simulink library "ThermalNodeTHB"  (R2018b)
settings: Solver=ode45  StartTime=0.0  StopTime=10.0  RelTol=1e-3  EnableMultiTasking=on
libraries: carnot x2
settings Model: Creator=Hafner  LastModifiedBy=drhf
settings DataIOCC: LimitDataPoints=on  SaveFormat=Array  SignalLoggingSaveFormat=ModelDataLogs
settings OptimizationCC: ExpressionDepthLimit=2147483647  LifeSpan=inf
settings DebuggingCC: UnderspecifiedInitializationDetection=Classic  MergeDetectMultiDrivingBlocksExec=none  SolverPrmCheckMsg=warning  FcnCallInpInsideContextMsg=warning  StateNameClashWarn=warning  SFUnexpectedBacktrackingDiag=warning  SFNoUnconditionalDefaultTransitionDiag=warning  SFExecutionAtInitializationDiag=none
settings HardwareCC: ProdBitPerPointer=32  ProdBitPerSizeT=32  ProdBitPerPtrDiffT=32  ProdLargestAtomicFloat=None  ProdIntDivRoundTo=Undefined  ProdEndianess=Unspecified  ProdWordSize=32  ProdHWDeviceType=32-bit Generic
settings ModelReferenceCC: PropagateSignalLabelsOutOfModel=off
settings SFSimCC: SimUseLocalCustomCode=off
settings RTWCC: RTWUseLocalCustomCode=off
settings CodeAppCC: StateflowObjectComments=on
settings GRTTargetCC: TargetLangStandard=C89/C90 (ANSI)  GeneratePreprocessorConditionals=Disable all  CombineOutputUpdateFcns=off  GRTInterface=on
settings ConfigComp: CovMetricSettings=dw  CovHtmlReporting=on  CovSaveCumulativeToWorkspaceVar=on  CovSaveSingleToWorkspaceVar=on  CovExternalEMLEnable=off

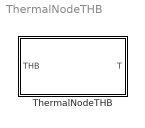
== system ThermalNodeTHB ==
  ThermalNodeTHB : Subsystem  mask(Thermal Node){UA=1, mcp=4182, Tini=20}
      mask prompts: UA "UA: thermal loss coefficient in W/K"; mcp "mcp: thermal capacity of the node in J/K"; Tini "Ambient temperature for losses (and initial Temp.) in °C"
      mask help: Thermal node with the THB as input.
      mask Help: web(fullfile(path_carnot('help'),'Thermal_Node.html'),'-helpbrowser')
      mask TypeOptions UA: Thermal_Node/UA
      mask TypeOptions mcp: Thermal_Node/mcp
      mask TypeOptions Tini: Tamb/Value
      mask Display: plot(-20,0,120,100,[10,70,70,10,10],[10,10,70,70,10],[70,90,90,30,10],[10,30,90,90,70],[90,70],[90,70],[50,30],[60,60],[40,40],[30,60])

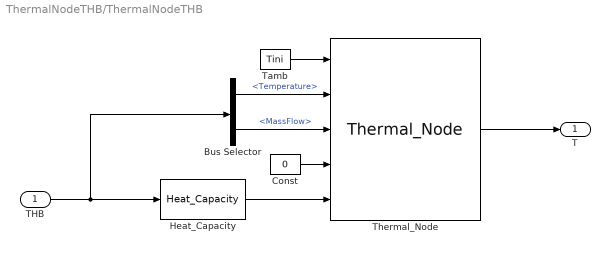
== system ThermalNodeTHB/ThermalNodeTHB ==
  THB : Inport
  Bus Selector : BusSelector  OutputSignals=Temperature,MassFlow
  Const : Constant  Value=0
  Heat_Capacity : carnot/Basic/Material_Properties/Heat_Capacity  VariantControl=CarlibClassic  INPUTARGUMENTS=THB  DEBUGLEVEL=DEBUGLEVEL  MAXTOTALWARNINGS=inf  MAXCONSECUTIVEWARNINGS=inf  WRITETOFILE=0  FILENAME='errors.txt'
      settings: SourceProductName=Carnot
  Tamb : Constant  Value=Tini
  Thermal_Node : carnot/Basic/Thermal_Models/Thermal_Node  UA=UA  mcp=mcp
      settings: SourceProductName=Carnot
  T : Outport  InitialOutput=20
  wires:
  Const/1 -> Thermal_Node/4
  Thermal_Node/1 -> T/1
  Bus Selector/1 -> Thermal_Node/2  "<Temperature>"
  Bus Selector/2 -> Thermal_Node/3  "<MassFlow>"
  THB/1 -> Bus Selector/1, Heat_Capacity/1
  Heat_Capacity/1 -> Thermal_Node/5
  Tamb/1 -> Thermal_Node/1
